simulink model "part02"  (R2023b)
settings: Solver=VariableStepAuto  StartTime=0.0  StopTime=1000  RelTol=1e-3
libraries: slctrl_linear x1, slpidlib x1, SignalEditorBlockLib x1
settings Model: Creator=UseR  LastModifiedBy=UseR

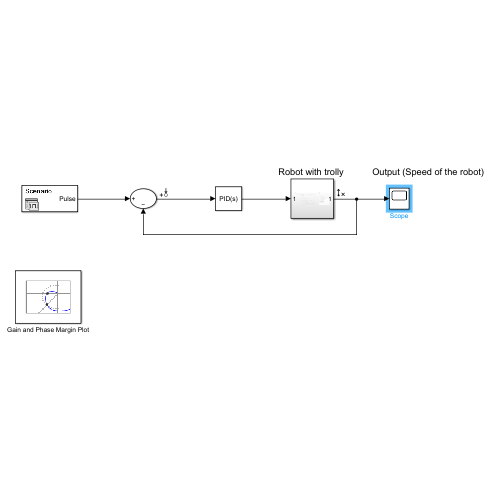
[thumbnail: Simulink's stored preview of the top-level diagram]
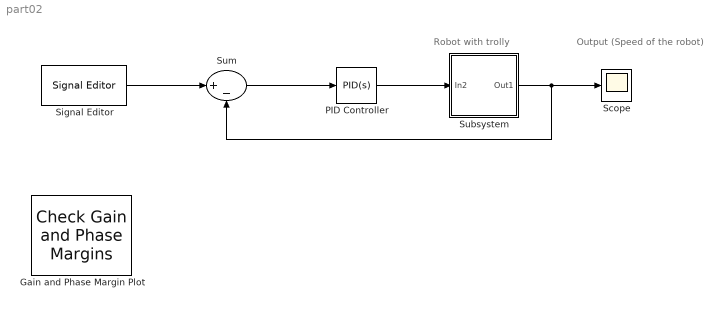
== system part02 ==
  note: Robot with trolly
  note: Output (Speed of the robot)
  Gain and Phase Margin Plot : slctrl_linear/Check Gain and Phase Margins  InstantiateOnLoad=on  SaveOperatingPoints=off  LinearizationIOs={'/Sum', 1, 'in', 'off', '';'/Subsystem', 1, 'out', 'on', ''}  LinearizeAt=SnapshotTimes  SnapshotTimes=[0]  TriggerType=rising  SampleTime=auto  RateConversionMethod=zoh  PreWarpFreq=10  UseExactDelayModel=off  UseFullBlockNameLabels=off  UseBusSignalLabels=off  enabled=on  stopWhenAssertionFail=off  export=off  ViewDlgPos=[538.6 196.2 509.6 389.6]  LaunchViewOnOpen=off  OpenViewOnLoad=off  FrequencyUnits=rad/s  MagnitudeUnits=dB  PhaseUnits=deg  TimeUnits=seconds  EnableMargins=off  GainMargin=[]  PhaseMargin=[]  PlotType=bode  FeedbackSign=-1
      settings: LibrarySourceBlock=slctrlblks/Linear Analysis Plots/Gain and Phase Margin Plot  SaveToWorkspace=off  SaveName=sys
  PID Controller : slpidlib/PID Controller  Controller=PID  Form=Parallel  TimeDomain=Continuous-time  UseExternalTs=off  SampleTime=-1  IntegratorMethod=Forward Euler  FilterMethod=Forward Euler  ControllerParametersSource=internal  P=1.11772359600471  I=1.55843985068434  UseKiTs=off  D=-1.42512019564477  N=0.833120453939515  UseFilter=on  TunerSelectOption=Transfer Function Based (PID Tuner App)  InitialConditionSource=internal  InitialConditionForIntegrator=0  InitialConditionForFilter=0  DifferentiatorICPrevScaledInput=0  ExternalReset=none  TrackingMode=off  Kt=1  LimitOutput=off  SatLimitsSource=internal  UpperSaturationLimit=inf  LowerSaturationLimit=-inf  LinearizeAsGain=on  AntiWindupMode=none  Kb=1  LimitIntegrator=off  UpperIntegratorSaturationLimit=inf  LowerIntegratorSaturationLimit=-inf  POutMin=[]  POutMax=[]  IOutMin=[]  IOutMax=[]  DOutMin=[]  DOutMax=[]  NOutMin=[]  NOutMax=[]  SumOutMin=[]  SumOutMax=[]  SaturationOutMin=[]  SaturationOutMax=[]  PParamMin=[]  PParamMax=[]  IParamMin=[]  IParamMax=[]  DParamMin=[]  DParamMax=[]  NParamMin=[]  NParamMax=[]  KbParamMin=[]  KbParamMax=[]  KtParamMin=[]  KtParamMax=[]  KbOutMin=[]  KbOutMax=[]  KtOutMin=[]  KtOutMax=[]  IntegratorOutMin=[]  IntegratorOutMax=[]  FilterOutMin=[]  FilterOutMax=[]  SumI1OutMin=[]  SumI1OutMax=[]  SumI2OutMin=[]  SumI2OutMax=[]  SumI3OutMin=[]  SumI3OutMax=[]  SumI4OutMin=[]  SumI4OutMax=[]  SumDOutMin=[]  SumDOutMax=[]  DifferentiatorOutMin=[]  DifferentiatorOutMax=[]  FilterDiffOutCoefMin=[]  FilterDiffOutCoefMax=[]  ReciprocalOutMin=[]  ReciprocalOutMax=[]  SumDenOutMin=[]  SumDenOutMax=[]  SumNumOutMin=[]  SumNumOutMax=[]  DivideOutMin=[]  DivideOutMax=[]  UdiffTsProdOutMin=[]  UdiffTsProdOutMax=[]  NTsProdOutMin=[]  NTsProdOutMax=[]  UintegralTsProdOutMin=[]  UintegralTsProdOutMax=[]  UngainTsProdOutMin=[]  UngainTsProdOutMax=[]  ClampingZeroOutDataTypeStr=Inherit: Inherit via back propagation  ClampingZeroOutMin=[]  ClampingZeroOutMax=[]  FilterDenConstantOutDataTypeStr=Inherit: Inherit via back propagation  FilterDenConstantOutMin=[]  FilterDenConstantOutMax=[]  PCopyOutDataTypeStr=Inherit: Inherit via back propagation  PCopyOutMin=[]  PCopyOutMax=[]  NCopyOutDataTypeStr=Inherit: Inherit via back propagation  NCopyOutMin=[]  NCopyOutMax=[]  IntegratorContinuousStateAttributes=''  IntegratorStateMustResolveToSignalObject=off  IntegratorRTWStateStorageClass=Auto  FilterContinuousStateAttributes=''  FilterStateMustResolveToSignalObject=off  FilterRTWStateStorageClass=Auto  ParallelPVariant=InternalParameters  IdealPVariant=Disabled  IVariant=InternalParameters  DVariant=InternalParameters  IntegratorVariant=Continuous  SatVariant=Disabled  AWVariant=Passthrough  PCopyVariant=Disabled  TRVariant=Disabled  FdbkBlocksVariant=Forward  IdealPFdbkVariant=Disabled  SatFdbkVariant=Disabled  DerivativeFilterVariant=ContFilter  NVariant=InternalParameters  NCopyVariant=Disabled  FilterICVariant=InternalICsFilter  IntegratorICVariant=InternalICs  ExternalResetVariant=Disabled  TRSumVariant=Passthrough  SumFdbkVariant=Disabled  SumVariant=Sum_PID  TsampFilterVariant=InternalTs  TsampNgainVariant=Passthrough  TsampIntegralVariant=Disabled_SignalSpec  ExternalSaturationOutDataTypeStr=Inherit: Same as second input
  Scope : Scope
  Signal Editor : SignalEditorBlockLib/Signal Editor  FileName=C:\Users\UseR\OneDrive\Desktop\untitled.mat  ActiveScenario=Scenario  ActiveSignal=Pulse  IsBus=off  OutputBusObjectStr=Bus: BusObject  SampleTime=0  Interpolate=off  ZeroCross=off  OutputAfterFinalValue=Setting to zero  Unit=inherit  PreserveSignalName=on  ApplySigPropsToAllScenarios=on  ApplySigPropsToAllSignals=off
  Subsystem : Subsystem
  Sum : Sum  Inputs=|+-
  wires:
  Subsystem/1(Out1) -> Scope/1, Sum/2
  Signal Editor/1 -> Sum/1
  Sum/1 -> PID Controller/1
  PID Controller/1 -> Subsystem/1(In2)

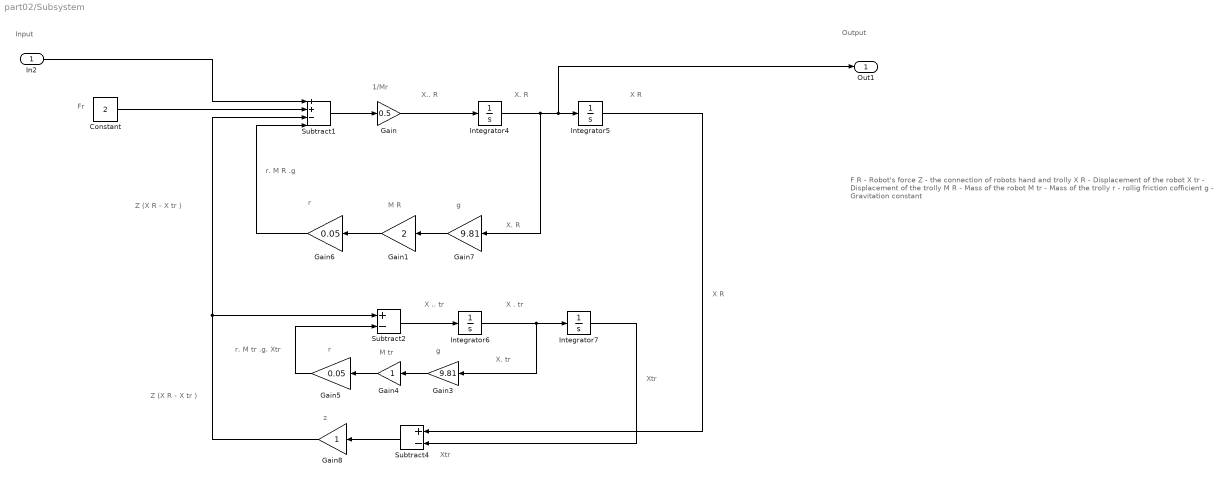
== system part02/Subsystem ==
  note: M tr
  note: g
  note: Xtr
  note: X .. tr
  note: Xtr
  note: r
  note: z
  note: r. M R .g
  note: r. M tr .g. Xtr
  note: r
  note: Z (X R - X tr )
  note: X. R
  note: X. R
  note: X. tr
  note: 1/Mr
  note: X . tr
  note: X.. R
  note: Fr
  note: M R
  note: X R
  note: X R
  note: g
  note: Input
  note: Output
  note: Z (X R - X tr )
  note: F R - Robot's force
      |
      | Z - the connection of robots hand and trolly
      |
      | X R - Displacement of the robot
      |
      | X tr - Displacement of the trolly
      |
      | M R - Mass of the robot
      |
      | M tr - Mass of the trolly
      |
      | r - rollig friction cofficient
      |
      | g - Gravitation constant
  In2 : Inport
  Constant : Constant  Value=2
  Gain : Gain  Gain=0.5
  Gain1 : Gain  Gain=2
  Gain3 : Gain  Gain=9.81
  Gain4 : Gain
  Gain5 : Gain  Gain=0.05
  Gain6 : Gain  Gain=0.05
  Gain7 : Gain  Gain=9.81
  Gain8 : Gain
  Integrator{4..7} (4 alike) : Integrator
  Subtract1 : Sum  Inputs=++--
  Subtract2 : Sum  Inputs=+-
  Subtract4 : Sum  Inputs=+-
  Out1 : Outport
  wires:
  Gain/1 -> Integrator4/1
  Integrator4/1 -> Integrator5/1, Out1/1, Gain7/1
  Subtract4/1 -> Gain8/1
  Gain8/1 -> Subtract1/3, Subtract2/1
  Constant/1 -> Subtract1/2
  Integrator5/1 -> Subtract4/1
  Gain7/1 -> Gain1/1
  In2/1 -> Subtract1/1
  Gain4/1 -> Gain5/1
  Subtract1/1 -> Gain/1
  Subtract2/1 -> Integrator6/1
  Gain1/1 -> Gain6/1
  Gain5/1 -> Subtract2/2
  Gain6/1 -> Subtract1/4
  Integrator6/1 -> Integrator7/1, Gain3/1
  Integrator7/1 -> Subtract4/2
  Gain3/1 -> Gain4/1
